simulink model "Optimal2Area_2Machine"  (R2022a)
settings: Solver=ode23  StartTime=0.0  StopTime=60  MaxStep=1e-3  RelTol=1e-3
values from neighbouring files (symbols this model uses):
  a12 = 1    [CallForSingleArea.m]    (also in Ricatti_CallForOptimal.m)
  b1 = 0.425    [CallForSingleArea.m]    (also in Ricatti_CallForOptimal.m)
  b2 = 0.425    [CallForSingleArea.m]    (also in Ricatti_CallForOptimal.m)
  Kps = 100    [CallForSingleArea.m]
  Ksg = 1    [CallForSingleArea.m]
  Kt = 1    [CallForSingleArea.m]
  PIT = 0.05    [CallForSingleArea.m]    (also in Ricatti_CallForOptimal.m)
  R = 3    [CallForSingleArea.m]
  Tps = 20    [CallForSingleArea.m]
  Tsg = 0.4    [CallForSingleArea.m]
  Tt = 0.5    [CallForSingleArea.m]
settings Model: Creator=ASUS  LastModifiedBy=ASUS

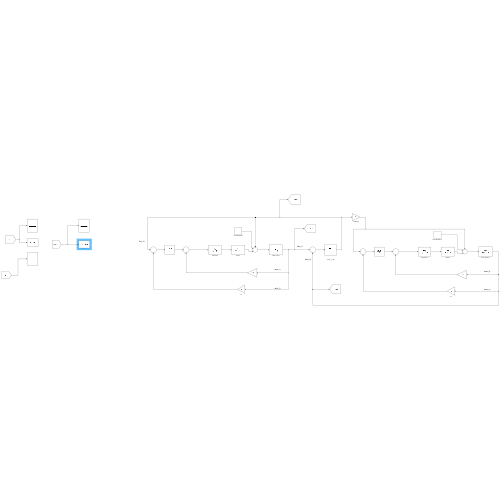
[thumbnail: Simulink's stored preview of the top-level diagram]
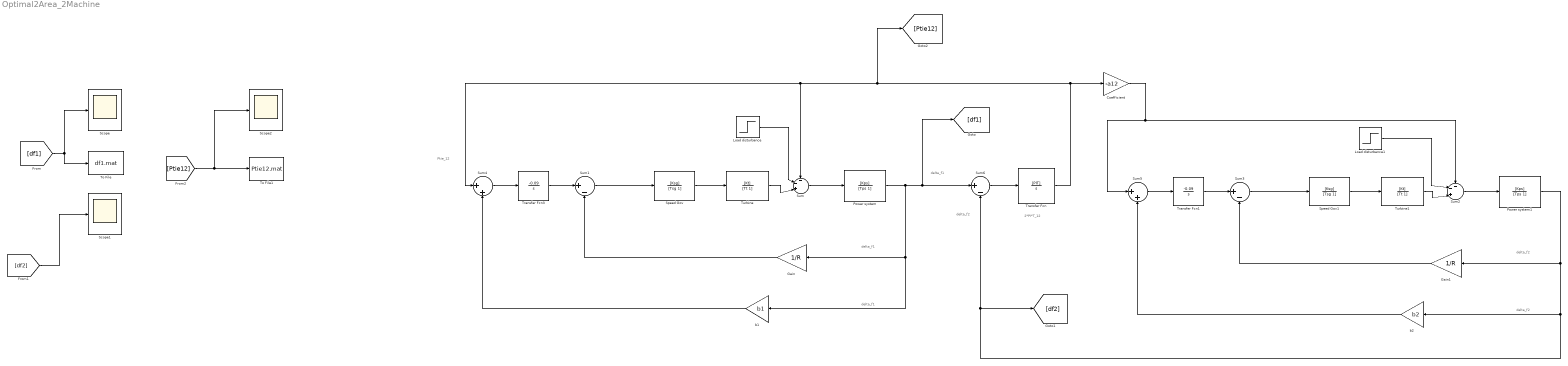
== system Optimal2Area_2Machine ==
  note: Ptie_12
  note: 2*PI*T_12
  note: delta_f1
  note: delta_f1
  note: delta_f2
  note: delta_f2
  note: delta_f1
  note: delta_f2
  " Speed Gov" : TransferFcn  Numerator=[Ksg]  Denominator=[Tsg 1]
  " Speed Gov1" : TransferFcn  Numerator=[Ksg]  Denominator=[Tsg 1]
  Coefficient : Gain  Gain=-a12
  Gain : Gain  Gain=1/R
  Gain1 : Gain  Gain=1/R
  Load disturbance : Step  Time=100  Before=0.01  After=0.01  SampleTime=0
  Load disturbance1 : Step  Time=100  After=0  SampleTime=0
  Power system : TransferFcn  Numerator=[Kps]  Denominator=[Tps 1]
  Power system1 : TransferFcn  Numerator=[Kps]  Denominator=[Tps 1]
  Scope : Scope
  Scope1 : Scope
  Scope2 : Scope
  Sum : Sum  Inputs=--+|
  Sum1 : Sum  Inputs=|+-
  Sum2 : Sum  Inputs=--+|
  Sum3 : Sum  Inputs=|+-
  Sum4 : Sum  Inputs=|++
  Sum5 : Sum  Inputs=|++
  Sum6 : Sum  Inputs=|+-
  To File : ToFile  Filename=df1.mat  MatrixName=df1
  To File1 : ToFile  Filename=Ptie12.mat  MatrixName=Ptie12
  Transfer Fcn : TransferFcn  Numerator=[PIT]  Denominator=[1 0]
  Transfer Fcn1 : TransferFcn  Numerator=[-0.09]  Denominator=[1 0]
  Transfer Fcn3 : TransferFcn  Numerator=[-0.09]  Denominator=[1 0]
  Turbine : TransferFcn  Numerator=[Kt]  Denominator=[Tt 1]
  Turbine1 : TransferFcn  Numerator=[Kt]  Denominator=[Tt 1]
  b1 : Gain  Gain=b1
  b2 : Gain  Gain=b2
  wires:
  Load disturbance/1 -> Sum/2
  Sum1/1 -> " Speed Gov"/1
  Power system/1 -> [df1], Sum6/1, b1/1, Gain/1
  Gain/1 -> Sum1/2
  Sum/1 -> Power system/1
  " Speed Gov"/1 -> Turbine/1
  Turbine/1 -> Sum/3
  b1/1 -> Sum4/2
  Sum4/1 -> Transfer Fcn3/1
  Transfer Fcn3/1 -> Sum1/1
  Transfer Fcn1/1 -> Sum3/1
  Sum5/1 -> Transfer Fcn1/1
  b2/1 -> Sum5/2
  Sum3/1 -> " Speed Gov1"/1
  Load disturbance1/1 -> Sum2/2
  " Speed Gov1"/1 -> Turbine1/1
  Sum2/1 -> Power system1/1
  Turbine1/1 -> Sum2/3
  Power system1/1 -> [df2], Sum6/2, b2/1, Gain1/1
  Gain1/1 -> Sum3/2
  Sum6/1 -> Transfer Fcn/1
  Transfer Fcn/1 -> Coefficient/1, [Ptie12], Sum/1, Sum4/1
  Coefficient/1 -> Sum2/1, Sum5/1
  [df1] -> To File/1, Scope/1
  [df2] -> Scope1/1
  [Ptie12] -> To File1/1, Scope2/1
